simulink model "motor_speed_controler"  (R2019a)
settings: Solver=odeN  StartTime=0.0  StopTime=600  MaxStep=Ts  RelTol=1e-1  AbsTol=1e-2  EnableMultiTasking=on
model workspace (MAT data in the model file):
  encoderResolution = 2000
  hallOffset = '0.5'
  indexOffset = 850
  polePairs = '4'
values from neighbouring files (symbols this model uses):
  alpha = 0    [parameters.m]
  Area = 1.13    [parameters.m]
  c_d = 0.5    [parameters.m]
  f = 0.018    [parameters.m]
  g = 9.81    [parameters.m]
  i_d = 3    [parameters.m]
  I_initial = v_desired/(R_bx)    (= 0)    [parameters.m]
  Jb = (m_b)*((R_bxb)^2)    (= 41.86125)    [parameters.m]
  Jx = (m_x)*((R_bx)^2)    (= 29.64574716)    [parameters.m]
  m_b = 450    [parameters.m]
  m_x = 159    [parameters.m]
  p = 1.204    [parameters.m]
  R_bx = 0.4318    [parameters.m]
  R_bxb = 0.305    [parameters.m]
  Ts = 1e-4    (= 0.0001)    [parameters.m]
undefined symbols (not defined in the file or in its folder): h, J_trans
libraries: fl_lib x42, nesl_utility x17, simulink x16, ee_lib x7, spsBreakerLib x6, spsThreePhaseParallelRLCLoadLib x4, spsSynchronousMachineSIFundamentalLib x4, spsThreePhaseSourceLib x2, spsCurrentMeasurementLib x2, sdl_lib x1, powerlib x1
(part 2 of 2)

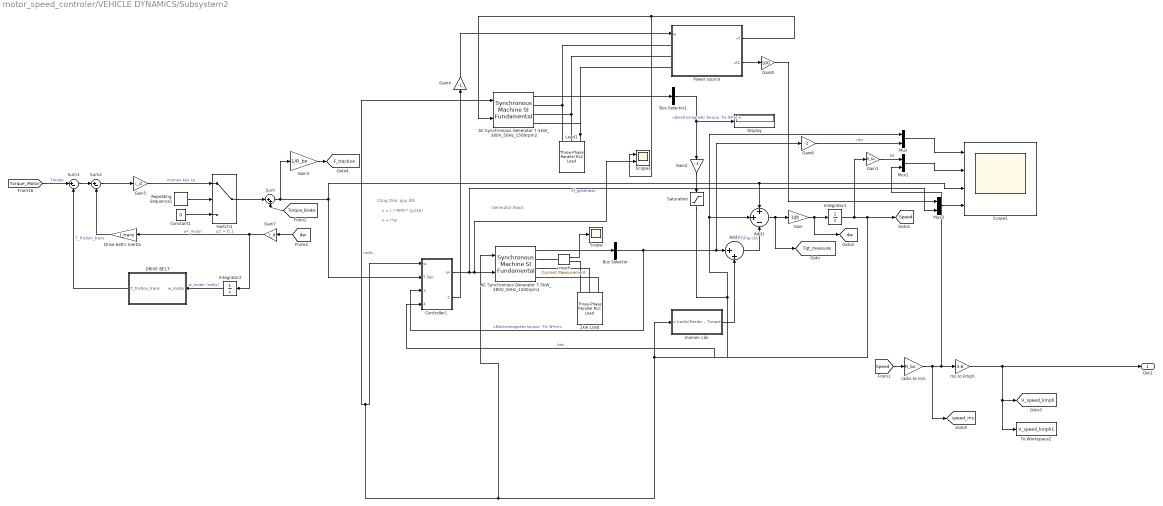
== system motor_speed_controler/VEHICLE DYNAMICS/Subsystem2 ==
  note: Công thức quy đổi
  note: v = r*w
  note: Generator Block
  note: v = r * RPM * (pi/30)
  2kw Load : spsThreePhaseParallelRLCLoadLib/Three-Phase Parallel RLC Load  LConnTagsString=A|B|C  Configuration=Y (grounded)  NominalVoltage=72  Vabc=[1e3 1e3 1e3]  Vabcp=[1e3 1e3 1e3]  NominalFrequency=50  UnbalancedPower=off  ActivePower=1000  InductivePower=0  CapacitivePower=0  Pabc=[10e3 9e3 11e3]  QLabc=[100 90 110]  QCabc=[100 90 110]  Pabcp=[10e3 9e3 11e3]  QLabcp=[100 90 110]  QCabcp=[100 90 110]  Measurements=None  LoadType=constant Z
      settings: SourceProductName=Simscape Electrical
  AC Synchronous Generator 7.5kW_380V_50Hz_1500rpm1 : spsSynchronousMachineSIFundamentalLib/Synchronous Machine SI Fundamental  PresetModel=No  MechanicalLoad=Speed w  ShowDetailedParameters=on  RotorType=Salient-pole  Units=SI fundamental parameters  MeasurementBus=off  NominalParameters=[7500 220 50 2]  Stator=[1.62 0.004527 0.1086 0.05175]  Field=[1.208 0.01132]  Dampers2=[ 0.0664, 1.387e-3, 0.0292, 6.896e-4, 7.907e-3, 2.477e-3]  Dampers1=[3.142 0.007334 4.772 0.01015]  Mechanical=[0.0923 0.009 2]  PolePairs=2  InitialConditions="[ 0  0  0  0  0  0  0  0 0]"  SetSaturation=off  Saturation=[695.64,774.7,917.5,1001.6,1082.2,1175.9,1293.6,1430.2,1583.7;9660,10623,12243,13063,13757,14437,15180,15890,16567]  DisplayVfd=off  LoadFlowParameters=[1,0,0,0,0]  TsPowergui=0  TsBlock=-1  IterativeModel=Trapezoidal non iterative  IterativeDiscreteModel=Trapezoidal non iterative  BusType=swing  Pref=0  Qref=0  Qmin=-inf  Qmax=inf  PLF=0  QLF=0
      settings: SourceProductName=Simscape Electrical  SourceProductBaseCode=PS
  AC Synchronous Generator 7.5kW_380V_50Hz_1500rpm2 : spsSynchronousMachineSIFundamentalLib/Synchronous Machine SI Fundamental  PresetModel=No  MechanicalLoad=Speed w  ShowDetailedParameters=on  RotorType=Salient-pole  Units=SI fundamental parameters  MeasurementBus=off  NominalParameters=[7500 220 50 2]  Stator=[1.62 0.004527 0.1086 0.05175]  Field=[1.208 0.01132]  Dampers2=[ 0.0664, 1.387e-3, 0.0292, 6.896e-4, 7.907e-3, 2.477e-3]  Dampers1=[3.142 0.007334 4.772 0.01015]  Mechanical=[0.0923 0.009 2]  PolePairs=2  InitialConditions="[ 0  0  0  0  0  0  0  0 0]"  SetSaturation=off  Saturation=[695.64,774.7,917.5,1001.6,1082.2,1175.9,1293.6,1430.2,1583.7;9660,10623,12243,13063,13757,14437,15180,15890,16567]  DisplayVfd=off  LoadFlowParameters=[1,0,0,0,0]  TsPowergui=0  TsBlock=-1  IterativeModel=Trapezoidal non iterative  IterativeDiscreteModel=Trapezoidal non iterative  BusType=swing  Pref=0  Qref=0  Qmin=-inf  Qmax=inf  PLF=0  QLF=0
      settings: SourceProductName=Simscape Electrical  SourceProductBaseCode=PS
  Add1 : Sum  Inputs=++-
  Add3 : Sum  Inputs=|++
  Bus Selector : BusSelector  OutputSignals="Mechanical.Electromagnetic torque  Te (N*m)"
  Bus Selector1 : BusSelector  OutputSignals="Mechanical.Electromagnetic torque  Te (N*m)"
  Constant1 : Constant  Value=0
  Controller1 : Subsystem
  DRIVE BELT : Subsystem
  Display : Display
  Drive belt's Inertia : Gain  Gain=J_trans
  Gain : Gain  Gain=1/Jb
  Gain1 : Gain  Gain=R_bx
  Gain2 : Gain  Gain=-1
  Gain3 : Gain  Gain=1/R_bx
  Gain4 : Gain  Gain=-1
  Gain5 : Gain  Gain=i_d
  Gain6 : Gain  Gain=-1
  Gain7 : Gain  Gain=i_d
  Gain8 : Gain  Gain=100
  Integrator1 : Integrator  InitialCondition=I_initial  LimitOutput=on  LowerSaturationLimit=0  ContinuousStateAttributes='velocity'
  Integrator2 : Integrator
  Load1 : spsThreePhaseParallelRLCLoadLib/Three-Phase Parallel RLC Load  LConnTagsString=A|B|C  Configuration=Y (grounded)  NominalVoltage=72  Vabc=[1e3 1e3 1e3]  Vabcp=[1e3 1e3 1e3]  NominalFrequency=50  UnbalancedPower=off  ActivePower=100  InductivePower=0  CapacitivePower=0  Pabc=[10e3 9e3 11e3]  QLabc=[100 90 110]  QCabc=[100 90 110]  Pabcp=[10e3 9e3 11e3]  QLabcp=[100 90 110]  QCabcp=[100 90 110]  Measurements=None  LoadType=constant Z
      settings: SourceProductName=Simscape Electrical
  Mux : Mux  Inputs=2
  Mux1 : Mux  Inputs=2
  Mux2 : Mux  Inputs=2
  Power source : Subsystem
  Repeating Sequence1 : simulink/Sources/Repeating Sequence  rep_seq_t=DriveCycle_time  rep_seq_y=DriveCycle_speed
  Saturation : Saturate  UpperLimit=inf  LowerLimit=0
  Scope : Scope
  Scope1 : Scope  NumInputPorts=4
  Scope3 : Scope  NumInputPorts=2
  Sum : Sum  Inputs=|++
  Sum1 : Sum  Inputs=|+-
  Sum2 : Sum  Inputs=|+-
  Switch1 : Switch  Criteria=u2 > Threshold  Threshold=0.1
  To Workspace2 : ToWorkspace  VariableName=V_speed_kmph1  SaveFormat=Structure With Time  SampleTime=-1
  i mach : spsCurrentMeasurementLib/Current Measurement  Tag=PoWeRsYsTeMmEaSuReMeNt  PhasorSimulation=off  OutputType=Magnitude  PSBequivalent=0
      settings: AttributesFormatString=\n  SourceProductName=Simscape Electrical
  momen cản : Subsystem
  ms to kmph : Gain  Gain=3.6
  rad/s to m/s : Gain  Gain=R_bx
  Out1 : Outport  VectorParamsAs1DForOutWhenUnconnected=on
  tag scope: F_tractive=global, Speed=global, Tqt_measure=global, V_speed_kmph=global, dw=global, speed_ms=global
  wires:
  Power source/2(vf1) -> Gain8/1
  Bus Selector1/1 -> Display/1, Gain2/1  "<Electromagnetic torque  Te (N*m)>"
  Repeating Sequence1/1 -> Switch1/2
  Integrator1/1 -> Gain1/1, [Speed], momen cản/1(v (rad/s)), AC Synchronous Generator 7.5kW_380V_50Hz_1500rpm1/1, AC Synchronous Generator 7.5kW_380V_50Hz_1500rpm2/1, Controller1/1(w)  "rad/s"
  Gain1/1 -> Mux1/1  "bệ"
  [Torque_Brake] -> Sum/2
  Sum2/1 -> Gain5/1
  Controller1/2(Vf_motor) -> Gain4/1
  Sum/1 -> Gain3/1, Controller1/2(T kéo), Scope1/3, Add1/1
  Switch1/1 -> Sum/1
  Controller1/1(Vf) -> Mux2/2, Scope3/2, AC Synchronous Generator 7.5kW_380V_50Hz_1500rpm1/2  "Vf_generator"
  Constant1/1 -> Switch1/3
  Integrator2/1 -> DRIVE BELT/1(w_motor)  "w_motor (rad/s)"
  Gain7/1 -> Integrator2/1, Drive belt's Inertia/1  "w*_motor"
  Mux2/1 -> Scope1/4
  Gain/1 -> [dw], Integrator1/1
  i mach/1 -> Scope/1
  Saturation/1 -> Controller1/4(T_motor), Mux/1, Add1/2  "kéo"
  Power source/1(vf) -> Scope3/1, AC Synchronous Generator 7.5kW_380V_50Hz_1500rpm2/2
  Bus Selector/1 -> Gain6/1, Add3/1, Controller1/3(T_measured)  "<Electromagnetic torque  Te (N*m)>"
  Add1/1 -> [Tqt_measure], Gain/1
  Gain2/1 -> Saturation/1
  Gain4/1 -> Power source/1(g)
  Add3/1 -> Add1/3  "Tổng cản"
  [Torque_Motor] -> Sum1/1  "Tmotor"
  Gain5/1 -> Switch1/1  "momen kéo xe"
  Gain8/1 -> Mux2/1
  Mux1/1 -> Scope1/2
  [Speed] -> rad/s to m/s/1
  Mux/1 -> Scope1/1
  AC Synchronous Generator 7.5kW_380V_50Hz_1500rpm1/1 -> Bus Selector/1
  AC Synchronous Generator 7.5kW_380V_50Hz_1500rpm2/1 -> Bus Selector1/1
  Gain6/1 -> Mux/2  "cản"
  Sum1/1 -> Sum2/1
  [dw] -> Gain7/1
  DRIVE BELT/1(T_friction_trans) -> Sum1/2  "T_friction_trans"
  Drive belt's Inertia/1 -> Sum2/2
  ms to kmph/1 -> Out1/1, To Workspace2/1, [V_speed_kmph]
  rad/s to m/s/1 -> [speed_ms], Mux1/2, ms to kmph/1
  momen cản/1(Resitive Torque) -> Add3/2
  Gain3/1 -> [F_tractive]
  connections:
  i mach/RConn1 -- 2kw Load/LConn1
  2kw Load/LConn3 -- AC Synchronous Generator 7.5kW_380V_50Hz_1500rpm1/RConn3
  Load1/LConn2 -- Power source/LConn2 -- AC Synchronous Generator 7.5kW_380V_50Hz_1500rpm2/RConn2
  Load1/LConn3 -- AC Synchronous Generator 7.5kW_380V_50Hz_1500rpm2/RConn3 -- Power source/LConn3
  Load1/LConn1 -- Power source/LConn1 -- AC Synchronous Generator 7.5kW_380V_50Hz_1500rpm2/RConn1
  AC Synchronous Generator 7.5kW_380V_50Hz_1500rpm1/RConn2 -- 2kw Load/LConn2
  AC Synchronous Generator 7.5kW_380V_50Hz_1500rpm1/RConn1 -- i mach/LConn1

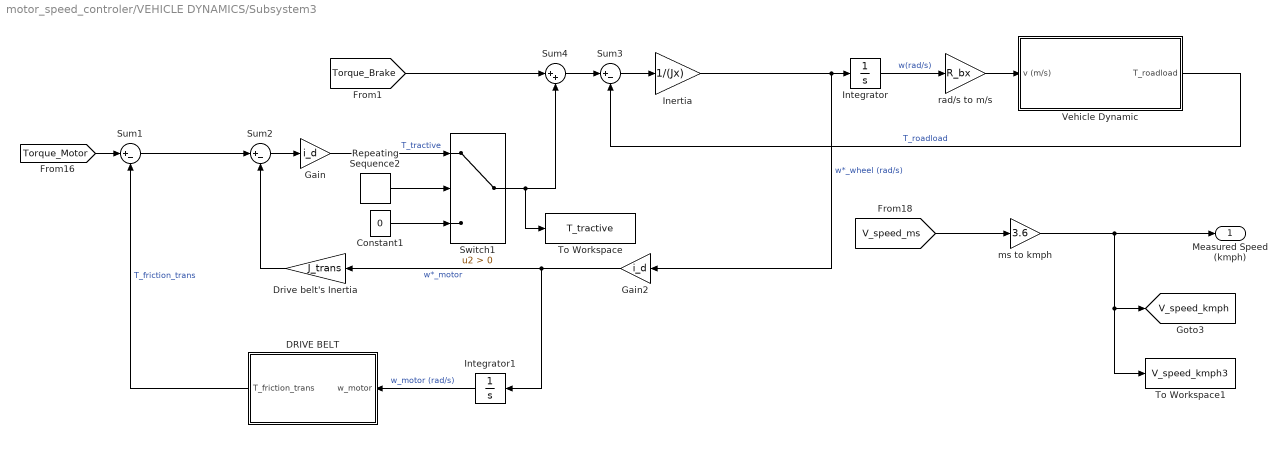
== system motor_speed_controler/VEHICLE DYNAMICS/Subsystem3 ==
  Constant1 : Constant  Value=0
  DRIVE BELT : Subsystem
  Drive belt's Inertia : Gain  Gain=J_trans
  Gain : Gain  Gain=i_d
  Gain2 : Gain  Gain=i_d
  Inertia : Gain  Gain=1/(Jx)
  Integrator : Integrator
  Integrator1 : Integrator
  Repeating Sequence2 : simulink/Sources/Repeating Sequence  rep_seq_t=DriveCycle_time  rep_seq_y=DriveCycle_speed
  Sum1 : Sum  Inputs=|+-
  Sum2 : Sum  Inputs=|+-
  Sum3 : Sum  Inputs=|+-
  Sum4 : Sum  Inputs=|++
  Switch1 : Switch  Criteria=u2 > Threshold
  To Workspace : ToWorkspace  VariableName=T_tractive  SaveFormat=Structure With Time  SampleTime=-1
  To Workspace1 : ToWorkspace  VariableName=V_speed_kmph3  SaveFormat=Structure With Time  SampleTime=-1
  Vehicle Dynamic : Subsystem
  ms to kmph : Gain  Gain=3.6
  rad/s to m/s : Gain  Gain=R_bx
  Measured Speed (kmph) : Outport  VectorParamsAs1DForOutWhenUnconnected=on
  tag scope: V_speed_kmph=global
  wires:
  Sum2/1 -> Gain/1
  DRIVE BELT/1(T_friction_trans) -> Sum1/2  "T_friction_trans"
  Inertia/1 -> Integrator/1, Gain2/1  "w*_wheel (rad/s)"
  Repeating Sequence2/1 -> Switch1/2
  [Torque_Brake] -> Sum4/1
  Gain2/1 -> Integrator1/1, Drive belt's Inertia/1  "w*_motor"
  Sum3/1 -> Inertia/1
  Vehicle Dynamic/1(T_roadload) -> Sum3/2  "T_roadload"
  Sum1/1 -> Sum2/1
  ms to kmph/1 -> Measured Speed (kmph)/1, To Workspace1/1, [V_speed_kmph]
  Drive belt's Inertia/1 -> Sum2/2
  [V_speed_ms] -> ms to kmph/1
  Integrator/1 -> rad/s to m/s/1  "w(rad/s)"
  rad/s to m/s/1 -> Vehicle Dynamic/1(v (m/s))
  Constant1/1 -> Switch1/3
  Sum4/1 -> Sum3/1
  [Torque_Motor] -> Sum1/1
  Switch1/1 -> Sum4/2, To Workspace/1
  Integrator1/1 -> DRIVE BELT/1(w_motor)  "w_motor (rad/s)"
  Gain/1 -> Switch1/1  "T_tractive"

== system motor_speed_controler/BLDC MOTOR DRIVER/Buck Converter/Sensing Vin ==
  PS-Simulink Converter4 : nesl_utility/PS-Simulink Converter  PhysicalDomain=network_engine_domain  SubClassName=ps_output  LeftPortType=input  RightPortType=output  PseudoPeriodic=off  Frequencies=[]  Unit=V  AffineConversion=off
      settings: SourceProductBaseCode=PW,SS
  Voltage Sensor : fl_lib/Electrical/Electrical Sensors/Voltage Sensor
  + : PMIOPort  Side=Left
  - : PMIOPort  Port=2  Side=Right
  tag scope: voltage_dc=global
  wires:
  PS-Simulink Converter4/1 -> [voltage_dc]
  connections:
  Voltage Sensor/LConn1 -- +/RConn1
  Voltage Sensor/RConn2 -- -/RConn1
  PS-Simulink Converter4/LConn1 -- Voltage Sensor/RConn1

== system motor_speed_controler/BLDC MOTOR DRIVER/Buck Converter/Sensing I1 ==
  Current Sensor : fl_lib/Electrical/Electrical Sensors/Current Sensor
  PS-Simulink Converter3 : nesl_utility/PS-Simulink Converter  PhysicalDomain=network_engine_domain  SubClassName=ps_output  LeftPortType=input  RightPortType=output  PseudoPeriodic=off  Frequencies=[]  Unit=A  AffineConversion=off
      settings: SourceProductBaseCode=PW,SS
  + : PMIOPort  Side=Left
  - : PMIOPort  Port=2  Side=Right
  tag scope: current_dc=global
  wires:
  PS-Simulink Converter3/1 -> [current_dc]
  connections:
  Current Sensor/RConn2 -- -/RConn1
  Current Sensor/LConn1 -- +/RConn1
  Current Sensor/RConn1 -- PS-Simulink Converter3/LConn1

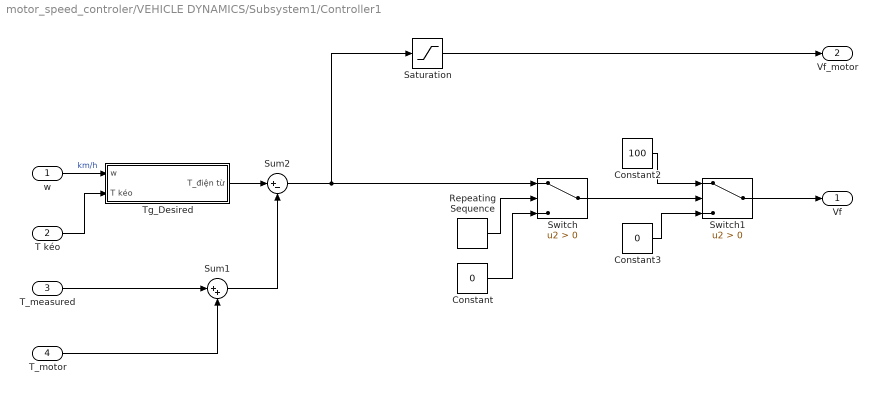
== system motor_speed_controler/VEHICLE DYNAMICS/Subsystem1/Controller1 ==
  w : Inport
  T kéo : Inport  Port=2
  T_measured : Inport  Port=3
  T_motor : Inport  Port=4
  Constant : Constant  Value=0
  Constant2 : Constant  Value=100
  Constant3 : Constant  Value=0
  Repeating Sequence : simulink/Sources/Repeating Sequence  rep_seq_t=DriveCycle_time  rep_seq_y=DriveCycle_speed
  Saturation : Saturate  UpperLimit=0  LowerLimit=-inf
  Sum1 : Sum  Inputs=|++
  Sum2 : Sum  Inputs=|+-
  Switch : Switch  Criteria=u2 > Threshold
  Switch1 : Switch  Criteria=u2 > Threshold
  Tg_Desired : Subsystem
  Vf : Outport
  Vf_motor : Outport  Port=2
  wires:
  Sum1/1 -> Sum2/2
  T_motor/1 -> Sum1/2
  T_measured/1 -> Sum1/1
  Sum2/1 -> Saturation/1, Switch/1
  Tg_Desired/1(T_điện từ) -> Sum2/1
  Switch1/1 -> Vf/1
  Constant3/1 -> Switch1/3
  Constant2/1 -> Switch1/1
  T kéo/1 -> Tg_Desired/2(T kéo)
  w/1 -> Tg_Desired/1(w)  "km/h"
  Constant/1 -> Switch/3
  Switch/1 -> Switch1/2
  Repeating Sequence/1 -> Switch/2
  Saturation/1 -> Vf_motor/1

== system motor_speed_controler/VEHICLE DYNAMICS/Subsystem1/DRIVE BELT ==
  w_motor : Inport
  Gain : Gain  Gain=0
  T_friction_trans : Outport  VectorParamsAs1DForOutWhenUnconnected=on
  tag scope: w_motor=global
  wires:
  w_motor/1 -> [w_motor], Gain/1
  Gain/1 -> T_friction_trans/1

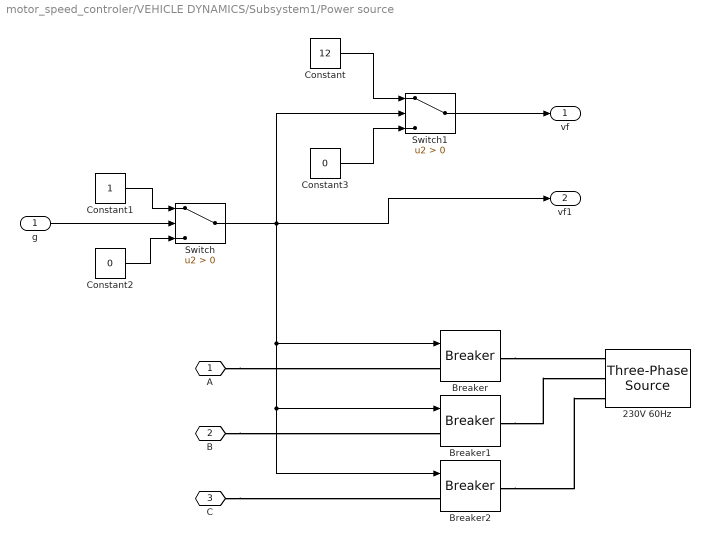
== system motor_speed_controler/VEHICLE DYNAMICS/Subsystem1/Power source ==
  g : Inport
  230V 60Hz : spsThreePhaseSourceLib/Three-Phase Source  InternalConnection=Yg  VoltagePhases=off  Voltage=72  PhaseAngle=0  Voltage_phases=[25e3 25e3 25e3]/sqrt(3)  PhaseAngles_phases=[0 -120 +120]  Frequency=50  NonIdealSource=on  SpecifyImpedance=off  Resistance=0.0002  Inductance=0.05e-3  ShortCircuitLevel=100e6  BaseVoltage=72  XRratio=7  BusType=swing  Pref=0  Qref=0  Prefabc=[10e3, 10e3, 10e3]  Qrefabc=[0, 0, 0]  Qmin=-inf  Qmax=inf
  Breaker : spsBreakerLib/Breaker  InitialState=0  SwitchingTimes="[1/60  5/60]"  External=on  BreakerResistance=0.01  SnubberResistance=1e6  SnubberCapacitance=inf  Measurements=None  MoreParameters=on  NoBreakLoop=off
      settings: SourceProductName=Simscape Electrical  SourceProductBaseCode=PS
  Breaker1 : spsBreakerLib/Breaker  InitialState=0  SwitchingTimes="[1/60  5/60]"  External=on  BreakerResistance=0.01  SnubberResistance=1e6  SnubberCapacitance=inf  Measurements=None  MoreParameters=on  NoBreakLoop=off
      settings: SourceProductName=Simscape Electrical  SourceProductBaseCode=PS
  Breaker2 : spsBreakerLib/Breaker  InitialState=0  SwitchingTimes="[1/60  5/60]"  External=on  BreakerResistance=0.01  SnubberResistance=1e6  SnubberCapacitance=inf  Measurements=None  MoreParameters=on  NoBreakLoop=off
      settings: SourceProductName=Simscape Electrical  SourceProductBaseCode=PS
  Constant : Constant  Value=12
  Constant1 : Constant
  Constant2 : Constant  Value=0
  Constant3 : Constant  Value=0
  Switch : Switch  Criteria=u2 > Threshold
  Switch1 : Switch  Criteria=u2 > Threshold
  A : PMIOPort  Side=Left
  B : PMIOPort  Port=2  Side=Left
  C : PMIOPort  Port=3  Side=Left
  vf : Outport
  vf1 : Outport  Port=2
  wires:
  Switch1/1 -> vf/1
  Constant3/1 -> Switch1/3
  Constant/1 -> Switch1/1
  g/1 -> Switch/2
  Constant2/1 -> Switch/3
  Constant1/1 -> Switch/1
  Switch/1 -> vf1/1, Switch1/2, Breaker/1, Breaker1/1, Breaker2/1
  connections:
  B/RConn1 -- Breaker1/LConn1
  C/RConn1 -- Breaker2/LConn1
  A/RConn1 -- Breaker/LConn1
  Breaker1/RConn1 -- 230V 60Hz/RConn2
  Breaker/RConn1 -- 230V 60Hz/RConn1
  Breaker2/RConn1 -- 230V 60Hz/RConn3

== system motor_speed_controler/VEHICLE DYNAMICS/Subsystem1/momen cản ==
  note: Total F_c = F_rolling + F_aerodynamics
  note: F_rolling = f*m_x*g*cos(alpha)
  note: F_aerodynamics = (1/2)*p*(c_d)*Area*(v^2)
  note: Phương trình lực cản
  v (rad/s) : Inport
  Add : Sum
  Constant : Constant  Value=0
  F_Rolling : Subsystem
  F_aerodynamics : Subsystem
  Gain : Gain  Gain=R_bx
  Gain1 : Gain  Gain=R_bx
  Gain2 : Gain  Gain=1/10
  Repeating Sequence : simulink/Sources/Repeating Sequence  rep_seq_t=DriveCycle_time  rep_seq_y=DriveCycle_speed
  Switch : Switch  Criteria=u2 > Threshold  Threshold=0.1
  Resitive Torque : Outport
  wires:
  F_aerodynamics/1(F_aero) -> Add/2
  v (rad/s)/1 -> Gain/1
  Add/1 -> Gain1/1
  Gain1/1 -> Gain2/1
  Gain/1 -> F_aerodynamics/1(v (m/s))
  Repeating Sequence/1 -> Switch/2  "km/h"
  Constant/1 -> Switch/3
  F_Rolling/1(F_rolling) -> Switch/1
  Switch/1 -> Add/1
  Gain2/1 -> Resitive Torque/1

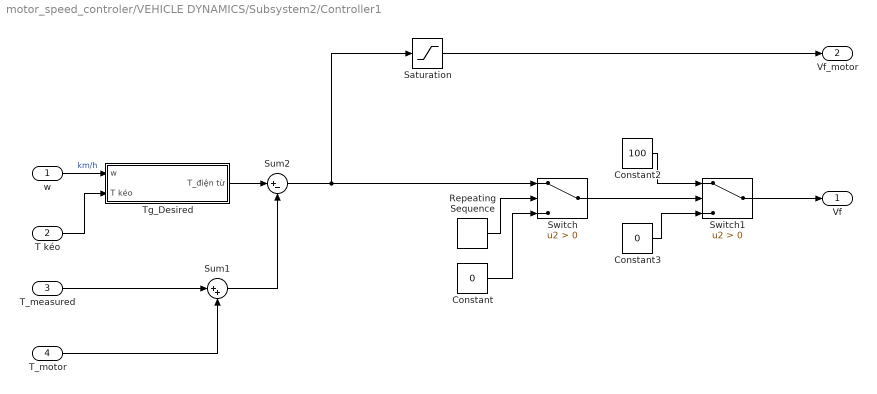
== system motor_speed_controler/VEHICLE DYNAMICS/Subsystem2/Controller1 ==
  w : Inport
  T kéo : Inport  Port=2
  T_measured : Inport  Port=3
  T_motor : Inport  Port=4
  Constant : Constant  Value=0
  Constant2 : Constant  Value=100
  Constant3 : Constant  Value=0
  Repeating Sequence : simulink/Sources/Repeating Sequence  rep_seq_t=DriveCycle_time  rep_seq_y=DriveCycle_speed
  Saturation : Saturate  UpperLimit=0  LowerLimit=-inf
  Sum1 : Sum  Inputs=|++
  Sum2 : Sum  Inputs=|+-
  Switch : Switch  Criteria=u2 > Threshold
  Switch1 : Switch  Criteria=u2 > Threshold
  Tg_Desired : Subsystem
  Vf : Outport
  Vf_motor : Outport  Port=2
  wires:
  Sum1/1 -> Sum2/2
  T_motor/1 -> Sum1/2
  T_measured/1 -> Sum1/1
  Sum2/1 -> Saturation/1, Switch/1
  Tg_Desired/1(T_điện từ) -> Sum2/1
  Switch1/1 -> Vf/1
  Constant3/1 -> Switch1/3
  Constant2/1 -> Switch1/1
  T kéo/1 -> Tg_Desired/2(T kéo)
  w/1 -> Tg_Desired/1(w)  "km/h"
  Constant/1 -> Switch/3
  Switch/1 -> Switch1/2
  Repeating Sequence/1 -> Switch/2
  Saturation/1 -> Vf_motor/1

== system motor_speed_controler/VEHICLE DYNAMICS/Subsystem2/DRIVE BELT ==
  w_motor : Inport
  Gain : Gain  Gain=0
  T_friction_trans : Outport  VectorParamsAs1DForOutWhenUnconnected=on
  tag scope: w_motor=global
  wires:
  w_motor/1 -> [w_motor], Gain/1
  Gain/1 -> T_friction_trans/1

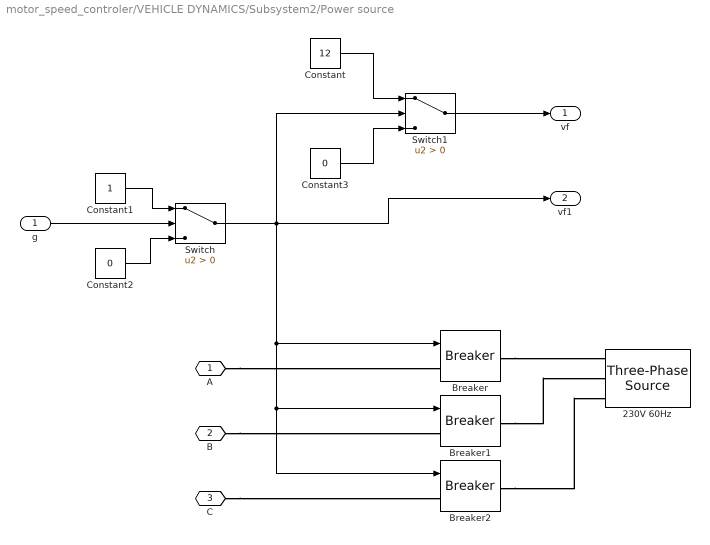
== system motor_speed_controler/VEHICLE DYNAMICS/Subsystem2/Power source ==
  g : Inport
  230V 60Hz : spsThreePhaseSourceLib/Three-Phase Source  InternalConnection=Yg  VoltagePhases=off  Voltage=72  PhaseAngle=0  Voltage_phases=[25e3 25e3 25e3]/sqrt(3)  PhaseAngles_phases=[0 -120 +120]  Frequency=50  NonIdealSource=on  SpecifyImpedance=off  Resistance=0.0002  Inductance=0.05e-3  ShortCircuitLevel=100e6  BaseVoltage=72  XRratio=7  BusType=swing  Pref=0  Qref=0  Prefabc=[10e3, 10e3, 10e3]  Qrefabc=[0, 0, 0]  Qmin=-inf  Qmax=inf
  Breaker : spsBreakerLib/Breaker  InitialState=0  SwitchingTimes="[1/60  5/60]"  External=on  BreakerResistance=0.01  SnubberResistance=1e6  SnubberCapacitance=inf  Measurements=None  MoreParameters=on  NoBreakLoop=off
      settings: SourceProductName=Simscape Electrical  SourceProductBaseCode=PS
  Breaker1 : spsBreakerLib/Breaker  InitialState=0  SwitchingTimes="[1/60  5/60]"  External=on  BreakerResistance=0.01  SnubberResistance=1e6  SnubberCapacitance=inf  Measurements=None  MoreParameters=on  NoBreakLoop=off
      settings: SourceProductName=Simscape Electrical  SourceProductBaseCode=PS
  Breaker2 : spsBreakerLib/Breaker  InitialState=0  SwitchingTimes="[1/60  5/60]"  External=on  BreakerResistance=0.01  SnubberResistance=1e6  SnubberCapacitance=inf  Measurements=None  MoreParameters=on  NoBreakLoop=off
      settings: SourceProductName=Simscape Electrical  SourceProductBaseCode=PS
  Constant : Constant  Value=12
  Constant1 : Constant
  Constant2 : Constant  Value=0
  Constant3 : Constant  Value=0
  Switch : Switch  Criteria=u2 > Threshold
  Switch1 : Switch  Criteria=u2 > Threshold
  A : PMIOPort  Side=Left
  B : PMIOPort  Port=2  Side=Left
  C : PMIOPort  Port=3  Side=Left
  vf : Outport
  vf1 : Outport  Port=2
  wires:
  Switch1/1 -> vf/1
  Constant3/1 -> Switch1/3
  Constant/1 -> Switch1/1
  g/1 -> Switch/2
  Constant2/1 -> Switch/3
  Constant1/1 -> Switch/1
  Switch/1 -> vf1/1, Switch1/2, Breaker/1, Breaker1/1, Breaker2/1
  connections:
  B/RConn1 -- Breaker1/LConn1
  C/RConn1 -- Breaker2/LConn1
  A/RConn1 -- Breaker/LConn1
  Breaker1/RConn1 -- 230V 60Hz/RConn2
  Breaker/RConn1 -- 230V 60Hz/RConn1
  Breaker2/RConn1 -- 230V 60Hz/RConn3

== system motor_speed_controler/VEHICLE DYNAMICS/Subsystem2/momen cản ==
  note: Total F_c = F_rolling + F_aerodynamics
  note: F_rolling = f*m_x*g*cos(alpha)
  note: F_aerodynamics = (1/2)*p*(c_d)*Area*(v^2)
  note: Phương trình lực cản
  v (rad/s) : Inport
  Add : Sum
  Constant : Constant  Value=0
  F_Rolling : Subsystem
  F_aerodynamics : Subsystem
  Gain : Gain  Gain=R_bx
  Gain1 : Gain  Gain=R_bx
  Gain2 : Gain  Gain=1/10
  Repeating Sequence : simulink/Sources/Repeating Sequence  rep_seq_t=DriveCycle_time  rep_seq_y=DriveCycle_speed
  Switch : Switch  Criteria=u2 > Threshold  Threshold=0.1
  Resitive Torque : Outport
  wires:
  F_aerodynamics/1(F_aero) -> Add/2
  v (rad/s)/1 -> Gain/1
  Add/1 -> Gain1/1
  Gain1/1 -> Gain2/1
  Gain/1 -> F_aerodynamics/1(v (m/s))
  Repeating Sequence/1 -> Switch/2  "km/h"
  Constant/1 -> Switch/3
  F_Rolling/1(F_rolling) -> Switch/1
  Switch/1 -> Add/1
  Gain2/1 -> Resitive Torque/1

== system motor_speed_controler/VEHICLE DYNAMICS/Subsystem3/DRIVE BELT ==
  w_motor : Inport
  Gain : Gain  Gain=0
  T_friction_trans : Outport  VectorParamsAs1DForOutWhenUnconnected=on
  tag scope: w_motor=global
  wires:
  w_motor/1 -> [w_motor], Gain/1
  Gain/1 -> T_friction_trans/1

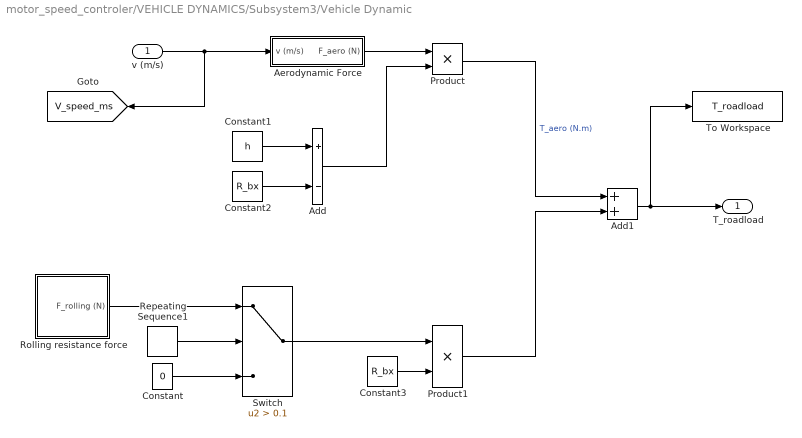
== system motor_speed_controler/VEHICLE DYNAMICS/Subsystem3/Vehicle Dynamic ==
  v (m/s) : Inport
  Add : Sum  Inputs=+-
  Add1 : Sum
  Aerodynamic Force : Subsystem
  Constant : Constant  Value=0
  Constant1 : Constant  Value=h
  Constant2 : Constant  Value=R_bx
  Constant3 : Constant  Value=R_bx
  Product : Product
  Product1 : Product
  Repeating Sequence1 : simulink/Sources/Repeating Sequence  rep_seq_t=DriveCycle_time  rep_seq_y=DriveCycle_speed
  Rolling resistance force : Subsystem
  Switch : Switch  Criteria=u2 > Threshold  Threshold=0.1
  To Workspace : ToWorkspace  VariableName=T_roadload  SaveFormat=Timeseries  SampleTime=-1
  T_roadload : Outport  VectorParamsAs1DForOutWhenUnconnected=on
  tag scope: V_speed_ms=global
  wires:
  Add1/1 -> To Workspace/1, T_roadload/1
  v (m/s)/1 -> [V_speed_ms], Aerodynamic Force/1(v (m/s))
  Aerodynamic Force/1(F_aero (N)) -> Product/1
  Constant/1 -> Switch/3
  Repeating Sequence1/1 -> Switch/2
  Rolling resistance force/1(F_rolling (N)) -> Switch/1
  Switch/1 -> Product1/1
  Constant1/1 -> Add/1
  Constant2/1 -> Add/2
  Add/1 -> Product/2
  Constant3/1 -> Product1/2
  Product1/1 -> Add1/2
  Product/1 -> Add1/1  "T_aero (N.m)"

== system motor_speed_controler/VEHICLE DYNAMICS/Subsystem1/Controller1/Tg_Desired ==
  w : Inport
  T kéo : Inport  Port=2
  Add : Sum  Inputs=|+-
  Add1 : Sum  Inputs=|++
  Add2 : Sum  Inputs=|+-
  Momen cản mong muốn : Subsystem
  Tqt mong muốn : Subsystem
  momen cản thực tế : Subsystem
  T_điện từ : Outport
  wires:
  momen cản thực tế/1(Resitive Torque) -> Add/2
  Add1/1 -> T_điện từ/1
  Momen cản mong muốn/1(T_road) -> Add/1
  w/1 -> momen cản thực tế/1(v (rad/s)), Momen cản mong muốn/1(rad/s)
  T kéo/1 -> Tqt mong muốn/1(Tk)
  Tqt mong muốn/1(Tqtx) -> Add2/1
  [Tqt_measure] -> Add2/2
  Add2/1 -> Add1/2
  Add/1 -> Add1/1

== system motor_speed_controler/VEHICLE DYNAMICS/Subsystem1/momen cản/F_Rolling ==
  Constant : Constant  Value=f
  Constant1 : Constant  Value=m_b
  Constant2 : Constant  Value=g
  Constant3 : Constant  Value=alpha
  Cos : Trigonometry  Operator=cos
  Product1 : Product  Inputs=4
  F_rolling : Outport
  wires:
  Constant2/1 -> Product1/3
  Constant3/1 -> Cos/1
  Product1/1 -> F_rolling/1
  Constant1/1 -> Product1/2
  Cos/1 -> Product1/4
  Constant/1 -> Product1/1

== system motor_speed_controler/VEHICLE DYNAMICS/Subsystem1/momen cản/F_aerodynamics ==
  v (m/s) : Inport
  Constant : Constant  Value=1/2
  Constant1 : Constant  Value=p
  Constant2 : Constant  Value=c_d
  Constant3 : Constant  Value=Area
  Product1 : Product  Inputs=5
  Square : Math  Operator=square  RndMeth=Zero  SaturateOnIntegerOverflow=on
  F_aero : Outport
  wires:
  Product1/1 -> F_aero/1
  Square/1 -> Product1/5  "v^2"
  Constant2/1 -> Product1/3
  Constant1/1 -> Product1/2
  Constant3/1 -> Product1/4
  Constant/1 -> Product1/1
  v (m/s)/1 -> Square/1

== system motor_speed_controler/VEHICLE DYNAMICS/Subsystem2/Controller1/Tg_Desired ==
  w : Inport
  T kéo : Inport  Port=2
  Add : Sum  Inputs=|+-
  Add1 : Sum  Inputs=|++
  Add2 : Sum  Inputs=|+-
  Momen cản mong muốn : Subsystem
  Tqt mong muốn : Subsystem
  momen cản thực tế : Subsystem
  T_điện từ : Outport
  wires:
  momen cản thực tế/1(Resitive Torque) -> Add/2
  Add1/1 -> T_điện từ/1
  Momen cản mong muốn/1(T_road) -> Add/1
  w/1 -> momen cản thực tế/1(v (rad/s)), Momen cản mong muốn/1(rad/s)
  T kéo/1 -> Tqt mong muốn/1(Tk)
  Tqt mong muốn/1(Tqtx) -> Add2/1
  [Tqt_measure] -> Add2/2
  Add2/1 -> Add1/2
  Add/1 -> Add1/1

== system motor_speed_controler/VEHICLE DYNAMICS/Subsystem2/momen cản/F_Rolling ==
  Constant : Constant  Value=f
  Constant1 : Constant  Value=m_b
  Constant2 : Constant  Value=g
  Constant3 : Constant  Value=alpha
  Cos : Trigonometry  Operator=cos
  Product1 : Product  Inputs=4
  F_rolling : Outport
  wires:
  Constant2/1 -> Product1/3
  Constant3/1 -> Cos/1
  Product1/1 -> F_rolling/1
  Constant1/1 -> Product1/2
  Cos/1 -> Product1/4
  Constant/1 -> Product1/1

== system motor_speed_controler/VEHICLE DYNAMICS/Subsystem2/momen cản/F_aerodynamics ==
  v (m/s) : Inport
  Constant : Constant  Value=1/2
  Constant1 : Constant  Value=p
  Constant2 : Constant  Value=c_d
  Constant3 : Constant  Value=Area
  Product1 : Product  Inputs=5
  Square : Math  Operator=square  RndMeth=Zero  SaturateOnIntegerOverflow=on
  F_aero : Outport
  wires:
  Product1/1 -> F_aero/1
  Square/1 -> Product1/5  "v^2"
  Constant2/1 -> Product1/3
  Constant1/1 -> Product1/2
  Constant3/1 -> Product1/4
  Constant/1 -> Product1/1
  v (m/s)/1 -> Square/1

== system motor_speed_controler/VEHICLE DYNAMICS/Subsystem3/Vehicle Dynamic/Aerodynamic Force ==
  v (m/s) : Inport
  Constant4 : Constant  Value=0.5
  Constant5 : Constant  Value=p
  Constant6 : Constant  Value=c_d
  Constant7 : Constant  Value=Area
  Math Function : Math  Operator=square  SaturateOnIntegerOverflow=on
  Product1 : Product  Inputs=5
  F_aero (N) : Outport  VectorParamsAs1DForOutWhenUnconnected=on
  wires:
  Constant6/1 -> Product1/2
  Math Function/1 -> Product1/5
  Constant7/1 -> Product1/1
  v (m/s)/1 -> Math Function/1
  Product1/1 -> F_aero (N)/1
  Constant4/1 -> Product1/4
  Constant5/1 -> Product1/3

== system motor_speed_controler/VEHICLE DYNAMICS/Subsystem3/Vehicle Dynamic/Rolling resistance force ==
  Constant : Constant  Value=f
  Constant1 : Constant  Value=m_x
  Constant2 : Constant  Value=g
  Constant3 : Constant  Value=alpha
  Cos : Trigonometry  Operator=cos
  Product : Product  Inputs=4
  F_rolling (N) : Outport  VectorParamsAs1DForOutWhenUnconnected=on
  wires:
  Constant3/1 -> Cos/1
  Constant1/1 -> Product/2
  Constant/1 -> Product/1
  Constant2/1 -> Product/3
  Cos/1 -> Product/4
  Product/1 -> F_rolling (N)/1

== system motor_speed_controler/VEHICLE DYNAMICS/Subsystem1/Controller1/Tg_Desired/Momen cản mong muốn ==
  rad/s : Inport
  Luc can : Subsystem
  R_bánh xe bệ2 : Gain  Gain=R_bxb
  R_bánh xe bệ3 : Gain  Gain=R_bxb
  T_road : Outport
  wires:
  Luc can/1(Resitive Force) -> R_bánh xe bệ3/1
  R_bánh xe bệ3/1 -> T_road/1
  R_bánh xe bệ2/1 -> Luc can/1(v)  "v (m/s)"
  rad/s/1 -> R_bánh xe bệ2/1

== system motor_speed_controler/VEHICLE DYNAMICS/Subsystem1/Controller1/Tg_Desired/Tqt mong muốn ==
  Tk : Inport
  Gain1 : Gain  Gain=1/Jx
  Integrator1 : Integrator  InitialCondition=I_initial  LimitOutput=on  LowerSaturationLimit=0  ContinuousStateAttributes='velocity'
  Sum1 : Sum  Inputs=|+-
  momen cản : Subsystem
  Tqtx : Outport
  wires:
  momen cản/1(Resitive Torque) -> Sum1/2  "Tc"
  Integrator1/1 -> momen cản/1(v (rad/s))  "v(rad/s)"
  Sum1/1 -> Tqtx/1, Gain1/1  "ma"
  Tk/1 -> Sum1/1
  Gain1/1 -> Integrator1/1  "dv/dt"

== system motor_speed_controler/VEHICLE DYNAMICS/Subsystem1/Controller1/Tg_Desired/momen cản thực tế ==
  note: Phương trình lực cản
  note: F_aerodynamics = (1/2)*p*(c_d)*Area*(v^2)
  note: F_rolling = f*m_x*g*cos(alpha)
  note: Total F_c = F_rolling + F_aerodynamics
  v (rad/s) : Inport
  Add : Sum
  Constant : Constant  Value=0
  F_Rolling : Subsystem
  F_aerodynamics : Subsystem
  Gain : Gain  Gain=R_bxb
  Gain1 : Gain  Gain=R_bxb
  Gain2 : Gain  Gain=1/10
  Repeating Sequence : simulink/Sources/Repeating Sequence  rep_seq_t=DriveCycle_time  rep_seq_y=DriveCycle_speed
  Switch : Switch  Criteria=u2 > Threshold  Threshold=0.1
  Resitive Torque : Outport
  wires:
  Gain1/1 -> Gain2/1
  Gain/1 -> F_aerodynamics/1(v (m/s))
  Add/1 -> Gain1/1
  v (rad/s)/1 -> Gain/1
  F_aerodynamics/1(F_aero) -> Add/2
  Gain2/1 -> Resitive Torque/1
  F_Rolling/1(F_rolling) -> Switch/1
  Repeating Sequence/1 -> Switch/2  "km/h"
  Constant/1 -> Switch/3
  Switch/1 -> Add/1

== system motor_speed_controler/VEHICLE DYNAMICS/Subsystem2/Controller1/Tg_Desired/Momen cản mong muốn ==
  rad/s : Inport
  Luc can : Subsystem
  R_bánh xe bệ2 : Gain  Gain=R_bxb
  R_bánh xe bệ3 : Gain  Gain=R_bxb
  T_road : Outport
  wires:
  Luc can/1(Resitive Force) -> R_bánh xe bệ3/1
  R_bánh xe bệ3/1 -> T_road/1
  R_bánh xe bệ2/1 -> Luc can/1(v)  "v (m/s)"
  rad/s/1 -> R_bánh xe bệ2/1

== system motor_speed_controler/VEHICLE DYNAMICS/Subsystem2/Controller1/Tg_Desired/Tqt mong muốn ==
  Tk : Inport
  Gain1 : Gain  Gain=1/Jx
  Integrator1 : Integrator  InitialCondition=I_initial  LimitOutput=on  LowerSaturationLimit=0  ContinuousStateAttributes='velocity'
  Sum1 : Sum  Inputs=|+-
  momen cản : Subsystem
  Tqtx : Outport
  wires:
  momen cản/1(Resitive Torque) -> Sum1/2  "Tc"
  Integrator1/1 -> momen cản/1(v (rad/s))  "v(rad/s)"
  Sum1/1 -> Tqtx/1, Gain1/1  "ma"
  Tk/1 -> Sum1/1
  Gain1/1 -> Integrator1/1  "dv/dt"

== system motor_speed_controler/VEHICLE DYNAMICS/Subsystem2/Controller1/Tg_Desired/momen cản thực tế ==
  note: Phương trình lực cản
  note: F_aerodynamics = (1/2)*p*(c_d)*Area*(v^2)
  note: F_rolling = f*m_x*g*cos(alpha)
  note: Total F_c = F_rolling + F_aerodynamics
  v (rad/s) : Inport
  Add : Sum
  Constant : Constant  Value=0
  F_Rolling : Subsystem
  F_aerodynamics : Subsystem
  Gain : Gain  Gain=R_bxb
  Gain1 : Gain  Gain=R_bxb
  Gain2 : Gain  Gain=1/10
  Repeating Sequence : simulink/Sources/Repeating Sequence  rep_seq_t=DriveCycle_time  rep_seq_y=DriveCycle_speed
  Switch : Switch  Criteria=u2 > Threshold  Threshold=0.1
  Resitive Torque : Outport
  wires:
  Gain1/1 -> Gain2/1
  Gain/1 -> F_aerodynamics/1(v (m/s))
  Add/1 -> Gain1/1
  v (rad/s)/1 -> Gain/1
  F_aerodynamics/1(F_aero) -> Add/2
  Gain2/1 -> Resitive Torque/1
  F_Rolling/1(F_rolling) -> Switch/1
  Repeating Sequence/1 -> Switch/2  "km/h"
  Constant/1 -> Switch/3
  Switch/1 -> Add/1

== system motor_speed_controler/VEHICLE DYNAMICS/Subsystem1/Controller1/Tg_Desired/Momen cản mong muốn/Luc can ==
  note: Total F_c = F_rolling + F_aerodynamics
  note: F_rolling = f*m_x*g*cos(alpha)
  note: F_aerodynamics = (1/2)*p*(c_d)*Area*(v^2)
  note: Phương trình lực cản
  v : Inport
  Add : Sum
  F_Rolling : Subsystem
  F_aerodynamics : Subsystem
  Resitive Force : Outport
  wires:
  F_aerodynamics/1(F_aero) -> Add/2
  Add/1 -> Resitive Force/1
  v/1 -> F_aerodynamics/1(v (m/s))
  F_Rolling/1(F_rolling) -> Add/1

== system motor_speed_controler/VEHICLE DYNAMICS/Subsystem1/Controller1/Tg_Desired/Tqt mong muốn/momen cản ==
  note: Total F_c = F_rolling + F_aerodynamics
  note: F_rolling = f*m_x*g*cos(alpha)
  note: F_aerodynamics = (1/2)*p*(c_d)*Area*(v^2)
  note: Phương trình lực cản
  v (rad/s) : Inport
  Add : Sum
  Constant : Constant  Value=0
  F_Rolling : Subsystem
  F_aerodynamics : Subsystem
  Gain : Gain  Gain=R_bx
  Gain1 : Gain  Gain=R_bx
  Repeating Sequence : simulink/Sources/Repeating Sequence  rep_seq_t=DriveCycle_time  rep_seq_y=DriveCycle_speed
  Switch : Switch  Criteria=u2 > Threshold  Threshold=0.1
  Resitive Torque : Outport
  wires:
  F_aerodynamics/1(F_aero) -> Add/2
  v (rad/s)/1 -> Gain/1
  Add/1 -> Gain1/1
  Gain1/1 -> Resitive Torque/1
  Gain/1 -> F_aerodynamics/1(v (m/s))
  Repeating Sequence/1 -> Switch/2  "km/h"
  Constant/1 -> Switch/3
  F_Rolling/1(F_rolling) -> Switch/1
  Switch/1 -> Add/1

== system motor_speed_controler/VEHICLE DYNAMICS/Subsystem1/Controller1/Tg_Desired/momen cản thực tế/F_Rolling ==
  Constant : Constant  Value=f
  Constant1 : Constant  Value=m_b
  Constant2 : Constant  Value=g
  Constant3 : Constant  Value=alpha
  Cos : Trigonometry  Operator=cos
  Product1 : Product  Inputs=4
  F_rolling : Outport
  wires:
  Constant2/1 -> Product1/3
  Constant3/1 -> Cos/1
  Product1/1 -> F_rolling/1
  Constant1/1 -> Product1/2
  Cos/1 -> Product1/4
  Constant/1 -> Product1/1

== system motor_speed_controler/VEHICLE DYNAMICS/Subsystem1/Controller1/Tg_Desired/momen cản thực tế/F_aerodynamics ==
  v (m/s) : Inport
  Constant : Constant  Value=1/2
  Constant1 : Constant  Value=p
  Constant2 : Constant  Value=c_d
  Constant3 : Constant  Value=Area
  Product1 : Product  Inputs=5
  Square : Math  Operator=square  RndMeth=Zero  SaturateOnIntegerOverflow=on
  F_aero : Outport
  wires:
  v (m/s)/1 -> Square/1
  Constant/1 -> Product1/1
  Constant3/1 -> Product1/4
  Constant1/1 -> Product1/2
  Constant2/1 -> Product1/3
  Square/1 -> Product1/5  "v^2"
  Product1/1 -> F_aero/1

== system motor_speed_controler/VEHICLE DYNAMICS/Subsystem2/Controller1/Tg_Desired/Momen cản mong muốn/Luc can ==
  note: Total F_c = F_rolling + F_aerodynamics
  note: F_rolling = f*m_x*g*cos(alpha)
  note: F_aerodynamics = (1/2)*p*(c_d)*Area*(v^2)
  note: Phương trình lực cản
  v : Inport
  Add : Sum
  F_Rolling : Subsystem
  F_aerodynamics : Subsystem
  Resitive Force : Outport
  wires:
  F_aerodynamics/1(F_aero) -> Add/2
  Add/1 -> Resitive Force/1
  v/1 -> F_aerodynamics/1(v (m/s))
  F_Rolling/1(F_rolling) -> Add/1

== system motor_speed_controler/VEHICLE DYNAMICS/Subsystem2/Controller1/Tg_Desired/Tqt mong muốn/momen cản ==
  note: Total F_c = F_rolling + F_aerodynamics
  note: F_rolling = f*m_x*g*cos(alpha)
  note: F_aerodynamics = (1/2)*p*(c_d)*Area*(v^2)
  note: Phương trình lực cản
  v (rad/s) : Inport
  Add : Sum
  Constant : Constant  Value=0
  F_Rolling : Subsystem
  F_aerodynamics : Subsystem
  Gain : Gain  Gain=R_bx
  Gain1 : Gain  Gain=R_bx
  Repeating Sequence : simulink/Sources/Repeating Sequence  rep_seq_t=DriveCycle_time  rep_seq_y=DriveCycle_speed
  Switch : Switch  Criteria=u2 > Threshold  Threshold=0.1
  Resitive Torque : Outport
  wires:
  F_aerodynamics/1(F_aero) -> Add/2
  v (rad/s)/1 -> Gain/1
  Add/1 -> Gain1/1
  Gain1/1 -> Resitive Torque/1
  Gain/1 -> F_aerodynamics/1(v (m/s))
  Repeating Sequence/1 -> Switch/2  "km/h"
  Constant/1 -> Switch/3
  F_Rolling/1(F_rolling) -> Switch/1
  Switch/1 -> Add/1

== system motor_speed_controler/VEHICLE DYNAMICS/Subsystem2/Controller1/Tg_Desired/momen cản thực tế/F_Rolling ==
  Constant : Constant  Value=f
  Constant1 : Constant  Value=m_b
  Constant2 : Constant  Value=g
  Constant3 : Constant  Value=alpha
  Cos : Trigonometry  Operator=cos
  Product1 : Product  Inputs=4
  F_rolling : Outport
  wires:
  Constant2/1 -> Product1/3
  Constant3/1 -> Cos/1
  Product1/1 -> F_rolling/1
  Constant1/1 -> Product1/2
  Cos/1 -> Product1/4
  Constant/1 -> Product1/1

== system motor_speed_controler/VEHICLE DYNAMICS/Subsystem2/Controller1/Tg_Desired/momen cản thực tế/F_aerodynamics ==
  v (m/s) : Inport
  Constant : Constant  Value=1/2
  Constant1 : Constant  Value=p
  Constant2 : Constant  Value=c_d
  Constant3 : Constant  Value=Area
  Product1 : Product  Inputs=5
  Square : Math  Operator=square  RndMeth=Zero  SaturateOnIntegerOverflow=on
  F_aero : Outport
  wires:
  v (m/s)/1 -> Square/1
  Constant/1 -> Product1/1
  Constant3/1 -> Product1/4
  Constant1/1 -> Product1/2
  Constant2/1 -> Product1/3
  Square/1 -> Product1/5  "v^2"
  Product1/1 -> F_aero/1

== system motor_speed_controler/VEHICLE DYNAMICS/Subsystem1/Controller1/Tg_Desired/Momen cản mong muốn/Luc can/F_Rolling ==
  Constant : Constant  Value=f
  Constant1 : Constant  Value=m_b
  Constant2 : Constant  Value=g
  Constant3 : Constant  Value=alpha
  Cos : Trigonometry  Operator=cos
  Product1 : Product  Inputs=4
  F_rolling : Outport
  wires:
  Constant2/1 -> Product1/3
  Constant3/1 -> Cos/1
  Product1/1 -> F_rolling/1
  Constant1/1 -> Product1/2
  Cos/1 -> Product1/4
  Constant/1 -> Product1/1

== system motor_speed_controler/VEHICLE DYNAMICS/Subsystem1/Controller1/Tg_Desired/Momen cản mong muốn/Luc can/F_aerodynamics ==
  v (m/s) : Inport
  Constant : Constant  Value=1/2
  Constant1 : Constant  Value=p
  Constant2 : Constant  Value=c_d
  Constant3 : Constant  Value=Area
  Product1 : Product  Inputs=5
  Square : Math  Operator=square  RndMeth=Zero  SaturateOnIntegerOverflow=on
  F_aero : Outport
  wires:
  Product1/1 -> F_aero/1
  Square/1 -> Product1/5  "v^2"
  Constant2/1 -> Product1/3
  Constant1/1 -> Product1/2
  Constant3/1 -> Product1/4
  Constant/1 -> Product1/1
  v (m/s)/1 -> Square/1

== system motor_speed_controler/VEHICLE DYNAMICS/Subsystem1/Controller1/Tg_Desired/Tqt mong muốn/momen cản/F_Rolling ==
  Constant : Constant  Value=f
  Constant1 : Constant  Value=m_b
  Constant2 : Constant  Value=g
  Constant3 : Constant  Value=alpha
  Cos : Trigonometry  Operator=cos
  Product1 : Product  Inputs=4
  F_rolling : Outport
  wires:
  Constant2/1 -> Product1/3
  Constant3/1 -> Cos/1
  Product1/1 -> F_rolling/1
  Constant1/1 -> Product1/2
  Cos/1 -> Product1/4
  Constant/1 -> Product1/1

== system motor_speed_controler/VEHICLE DYNAMICS/Subsystem1/Controller1/Tg_Desired/Tqt mong muốn/momen cản/F_aerodynamics ==
  v (m/s) : Inport
  Constant : Constant  Value=1/2
  Constant1 : Constant  Value=p
  Constant2 : Constant  Value=c_d
  Constant3 : Constant  Value=Area
  Product1 : Product  Inputs=5
  Square : Math  Operator=square  RndMeth=Zero  SaturateOnIntegerOverflow=on
  F_aero : Outport
  wires:
  Product1/1 -> F_aero/1
  Square/1 -> Product1/5  "v^2"
  Constant2/1 -> Product1/3
  Constant1/1 -> Product1/2
  Constant3/1 -> Product1/4
  Constant/1 -> Product1/1
  v (m/s)/1 -> Square/1

== system motor_speed_controler/VEHICLE DYNAMICS/Subsystem2/Controller1/Tg_Desired/Momen cản mong muốn/Luc can/F_Rolling ==
  Constant : Constant  Value=f
  Constant1 : Constant  Value=m_b
  Constant2 : Constant  Value=g
  Constant3 : Constant  Value=alpha
  Cos : Trigonometry  Operator=cos
  Product1 : Product  Inputs=4
  F_rolling : Outport
  wires:
  Constant2/1 -> Product1/3
  Constant3/1 -> Cos/1
  Product1/1 -> F_rolling/1
  Constant1/1 -> Product1/2
  Cos/1 -> Product1/4
  Constant/1 -> Product1/1

== system motor_speed_controler/VEHICLE DYNAMICS/Subsystem2/Controller1/Tg_Desired/Momen cản mong muốn/Luc can/F_aerodynamics ==
  v (m/s) : Inport
  Constant : Constant  Value=1/2
  Constant1 : Constant  Value=p
  Constant2 : Constant  Value=c_d
  Constant3 : Constant  Value=Area
  Product1 : Product  Inputs=5
  Square : Math  Operator=square  RndMeth=Zero  SaturateOnIntegerOverflow=on
  F_aero : Outport
  wires:
  Product1/1 -> F_aero/1
  Square/1 -> Product1/5  "v^2"
  Constant2/1 -> Product1/3
  Constant1/1 -> Product1/2
  Constant3/1 -> Product1/4
  Constant/1 -> Product1/1
  v (m/s)/1 -> Square/1

== system motor_speed_controler/VEHICLE DYNAMICS/Subsystem2/Controller1/Tg_Desired/Tqt mong muốn/momen cản/F_Rolling ==
  Constant : Constant  Value=f
  Constant1 : Constant  Value=m_b
  Constant2 : Constant  Value=g
  Constant3 : Constant  Value=alpha
  Cos : Trigonometry  Operator=cos
  Product1 : Product  Inputs=4
  F_rolling : Outport
  wires:
  Constant2/1 -> Product1/3
  Constant3/1 -> Cos/1
  Product1/1 -> F_rolling/1
  Constant1/1 -> Product1/2
  Cos/1 -> Product1/4
  Constant/1 -> Product1/1

== system motor_speed_controler/VEHICLE DYNAMICS/Subsystem2/Controller1/Tg_Desired/Tqt mong muốn/momen cản/F_aerodynamics ==
  v (m/s) : Inport
  Constant : Constant  Value=1/2
  Constant1 : Constant  Value=p
  Constant2 : Constant  Value=c_d
  Constant3 : Constant  Value=Area
  Product1 : Product  Inputs=5
  Square : Math  Operator=square  RndMeth=Zero  SaturateOnIntegerOverflow=on
  F_aero : Outport
  wires:
  Product1/1 -> F_aero/1
  Square/1 -> Product1/5  "v^2"
  Constant2/1 -> Product1/3
  Constant1/1 -> Product1/2
  Constant3/1 -> Product1/4
  Constant/1 -> Product1/1
  v (m/s)/1 -> Square/1
